simulink library "ACT_MAG"  (Simulink 9.0)
settings: Solver=VariableStepAuto  StartTime=0.0  StopTime=10.0  RelTol=1e-3
undefined symbols (not defined in the file): ACT_MAG
settings Model: SuppressorTable=22 serialization::archive 11 0 6 0 0 0 0 0  Creator=WilTravis  LastModifiedBy=WilTravis

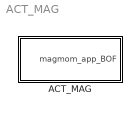
== system ACT_MAG ==
  ACT_MAG : Subsystem

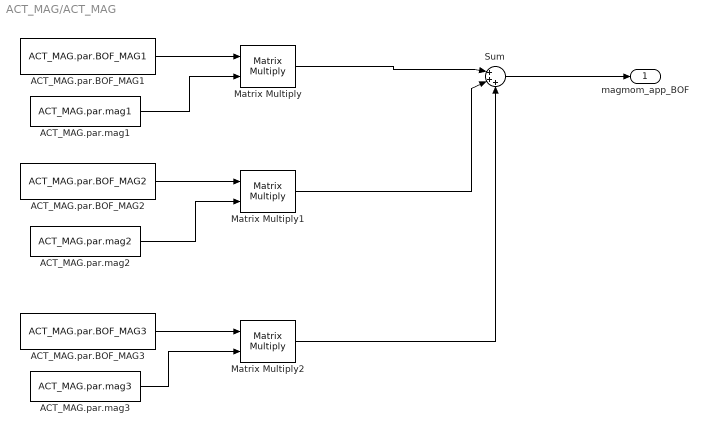
== system ACT_MAG/ACT_MAG ==
  ACT_MAG.par.BOF_MAG1 : Constant  Value=ACT_MAG.par.BOF_MAG1
  ACT_MAG.par.BOF_MAG2 : Constant  Value=ACT_MAG.par.BOF_MAG2
  ACT_MAG.par.BOF_MAG3 : Constant  Value=ACT_MAG.par.BOF_MAG3
  ACT_MAG.par.mag1 : Constant  Value=ACT_MAG.par.mag1
  "ACT_MAG.par.mag2 " : Constant  Value=ACT_MAG.par.mag2
  ACT_MAG.par.mag3 : Constant  Value=ACT_MAG.par.mag3
  Matrix Multiply : Product  Multiplication=Matrix(*)
  Matrix Multiply1 : Product  Multiplication=Matrix(*)
  Matrix Multiply2 : Product  Multiplication=Matrix(*)
  Sum : Sum  Inputs=|+++
  magmom_app_BOF : Outport
  wires:
  ACT_MAG.par.BOF_MAG2/1 -> Matrix Multiply1/1
  Matrix Multiply2/1 -> Sum/3
  "ACT_MAG.par.mag2 "/1 -> Matrix Multiply1/2
  ACT_MAG.par.mag3/1 -> Matrix Multiply2/2
  Sum/1 -> magmom_app_BOF/1
  ACT_MAG.par.BOF_MAG1/1 -> Matrix Multiply/1
  Matrix Multiply/1 -> Sum/1
  ACT_MAG.par.mag1/1 -> Matrix Multiply/2
  ACT_MAG.par.BOF_MAG3/1 -> Matrix Multiply2/1
  Matrix Multiply1/1 -> Sum/2
